simulink library "Collector_EN12975_CONF"  (R2013b)
settings: Solver=ode45  StartTime=0.0  StopTime=10.0  RelTol=1e-3
undefined symbols (not defined in the file): STC
libraries: carnot x2
settings Model: Creator=lena.frank  LastModifiedBy=drhf

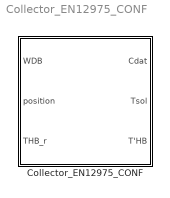
== system Collector_EN12975_CONF ==
  Collector_EN12975_CONF : Subsystem  mask(configurated Solar Thermal Collector){parameterfile=DefaultCollector, tini=20, Ncollector=1}
      mask prompts: parameterfile "Parameter set"; tini "Inital temperature in °C"; Ncollector "Number of collectors in parallel"
      mask help:
      | Dynamic 1-node collector model according to EN 12975 standard.
      | This block uses predefined parameter sets.
      mask init:
      | % path definitions
      | intpath = fullfile(path_carnot('intlibsl'), 'Source','Solar_Thermal', ...
      |     'Collector_EN12975_CONF','parameter_set');
      | pubpath = fullfile(path_carnot('libsl'), 'Source','Solar_Thermal', ...
      |     'Collector_EN12975_CONF','parameter_set');
      | 
      | [namelist, lib] = CarnotCallbacks_getConfNamelist(intpath,pubpath);
      | 
      | % set namelist in mask
      | if ~lib
      |     myMaskStylesVar{1} = ['popup(', namelist,')'];
      |     myMaskStylesVar{2} = 'edit';
      |     myMaskStylesVar{3} = 'edit';
      |     set_param(gcb, 'MaskStyles', myMaskStylesVar);
      | end
      | 
      | if exist(fullfile(intpath,[parameterfile '.mat']))
      |     load(fullfile(intpath,parameterfile));
      | else
      |     load(fullfile(pubpath,parameterfile));
      | end
      mask Help: web(fullfile(path_carnot('help'),'collector_en12975.html'),'-helpbrowser')
      mask TypeOptions parameterfile: DefaultCollector | Vitosol200F_SV2D_2_5m2 | Vitosol200T_SP2A_3m2 | Vitosol200T_SPE_1_6m2 | Vitosol200T_SPE_3_2m2 | Vitosol200T_SPL_200m2 | Vitosol300T_SP3B_3m2
      mask Display:
      | % user defined picture file
      | picfile = fullfile(path_carnot('intlibsl'), ...
      |     'Source','Solar_Thermal','Collector_EN12975_CONF','parameter_set', ...
      |      'Collector_CONF.jpg');
      | 
      | pic = false;
      | 
      | % show internal picture if defined
      | if ~BlockIsInCarnotLibrary    % if not located in library any more
      |     if exist(picfile)
      |         image(imread(picfile), [0, 0, 1, 1])
      |         set_param(gcb, 'BackgroundColor', 'White')
      |         pic = true;
      |     end
      | end
      | 
      | if ~pic    % show public picture
      |     disp('solar thermal\ncollector\nEN 12975\nIAM-Table')
      |     set_param(gcb, 'BackgroundColor', 'Yellow')
      | end
      | 
      | % Show port labels: same as port labels in the subsystem,
      | % but display with a picture covers the text. Have to reprint it.
      | port_label('input',1,'WDB')
      | port_label('input',2,'position')
      | port_label('input',3,'THB_r')
      | port_label('output',1,'Cdat')
      | port_label('output',2,'Tsol')
      | port_label('output',3,'THB_s')

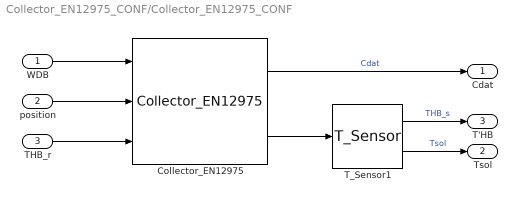
== system Collector_EN12975_CONF/Collector_EN12975_CONF ==
  WDB : Inport
  position : Inport  Port=2
  THB_r : Inport  Port=3
  Collector_EN12975 : carnot/Source/Solar_Thermal/Collector_EN12975  acol=STC.Acoll*Ncollector  len=STC.len  fta=STC.fta  c1=STC.c1  c2=STC.c2  c3=STC.c3  c4=STC.c4  c5=STC.c5  c6=STC.c6  kblangle=STC.KbAngles  KbL=STC.KbL  kbtangle=STC.KbAngles  KbT=STC.KbT  Kd=STC.Kd  lin=STC.lin/Ncollector  qua=STC.qua/(Ncollector^2)  tini=tini
  T_Sensor1 : carnot/Control/T_Sensor  tc=STC.SensorTimeConstant  t0=tini
  Cdat : Outport
  Tsol : Outport  Port=2
  T'HB : Outport  Port=3
  wires:
  Collector_EN12975/1 -> Cdat/1  "Cdat"
  THB_r/1 -> Collector_EN12975/3
  position/1 -> Collector_EN12975/2
  WDB/1 -> Collector_EN12975/1
  Collector_EN12975/2 -> T_Sensor1/1
  T_Sensor1/1 -> T'HB/1  "THB_s"
  T_Sensor1/2 -> Tsol/1  "Tsol"
